simulink model "Controls"  (R2024b)
settings: Solver=VariableStepAuto  StartTime=0.0  StopTime=10.0  RelTol=1e-3
settings Model: Creator=Rayhaan T  LastModifiedBy=Rayhaan T

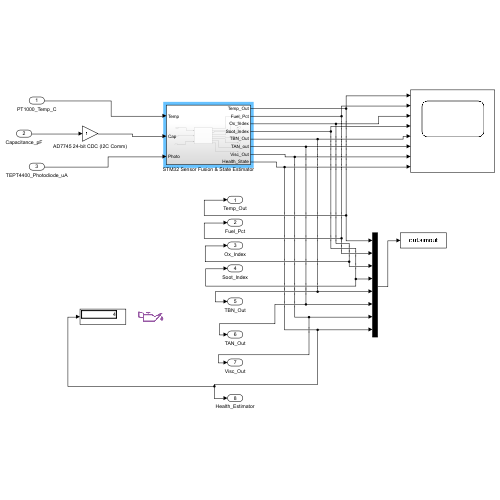
[thumbnail: Simulink's stored preview of the top-level diagram]
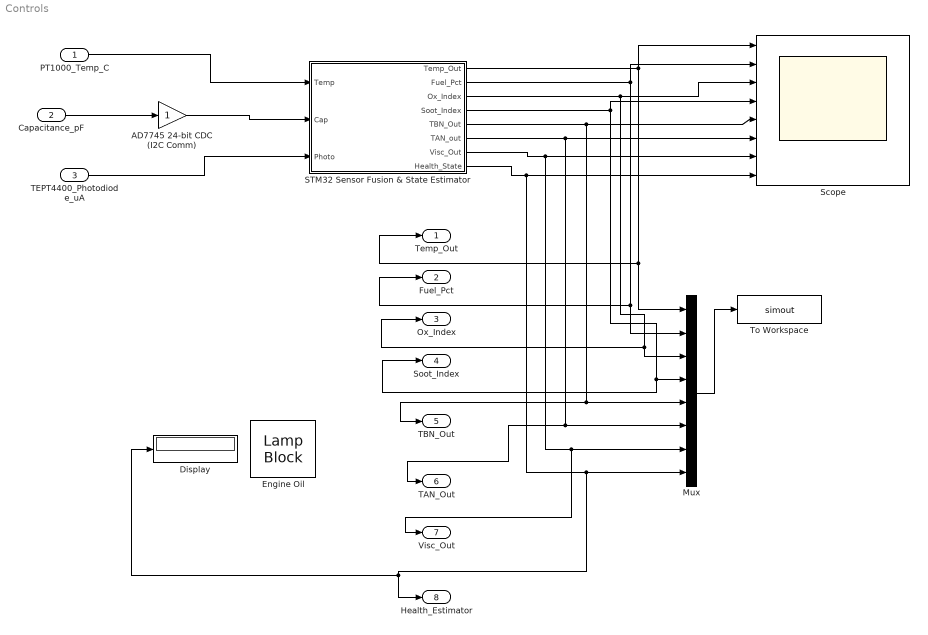
== system Controls ==
  PT1000_Temp_C : Inport
  Capacitance_pF : Inport  Port=2
  TEPT4400_Photodiode_uA : Inport  Port=3
  AD7745 24-bit CDC (I2C Comm) : Gain
  Display : Display
  Engine Oil : LampBlock  LabelPosition=Hide  Icon=EngineOil
  Mux : Mux  Inputs=8
  STM32 Sensor Fusion & State Estimator : Subsystem
  Scope : Scope  NumInputPorts=8
  To Workspace : ToWorkspace  VariableName=simout  SaveFormat=Timeseries  SampleTime=-1
  Temp_Out : Outport
  Fuel_Pct : Outport  Port=2
  Ox_Index : Outport  Port=3
  Soot_Index : Outport  Port=4
  TBN_Out : Outport  Port=5
  TAN_Out : Outport  Port=6
  Visc_Out : Outport  Port=7
  Health_Estimator : Outport  Port=8
  wires:
  Capacitance_pF/1 -> AD7745 24-bit CDC (I2C Comm)/1
  PT1000_Temp_C/1 -> STM32 Sensor Fusion & State Estimator/1(Temp)
  TEPT4400_Photodiode_uA/1 -> STM32 Sensor Fusion & State Estimator/3(Photo)
  STM32 Sensor Fusion & State Estimator/1(Temp_Out) -> Temp_Out/1, Mux/1, Scope/1
  STM32 Sensor Fusion & State Estimator/2(Fuel_Pct) -> Fuel_Pct/1, Mux/2, Scope/2
  STM32 Sensor Fusion & State Estimator/4(Soot_Index) -> Soot_Index/1, Mux/4, Scope/4
  STM32 Sensor Fusion & State Estimator/3(Ox_Index) -> Ox_Index/1, Mux/3, Scope/3
  AD7745 24-bit CDC (I2C Comm)/1 -> STM32 Sensor Fusion & State Estimator/2(Cap)
  Mux/1 -> To Workspace/1
  STM32 Sensor Fusion & State Estimator/5(TBN_Out) -> Mux/5, TBN_Out/1, Scope/5
  STM32 Sensor Fusion & State Estimator/6(TAN_out) -> Mux/6, TAN_Out/1, Scope/6
  STM32 Sensor Fusion & State Estimator/7(Visc_Out) -> Visc_Out/1, Mux/7, Scope/7
  STM32 Sensor Fusion & State Estimator/8(Health_State) -> Display/1, Health_Estimator/1, Mux/8, Scope/8

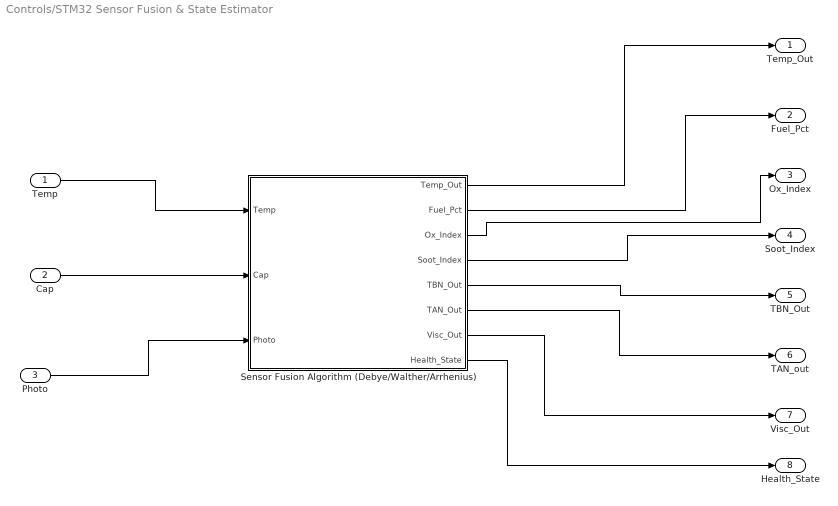
== system Controls/STM32 Sensor Fusion & State Estimator ==
  Temp : Inport
  Cap : Inport  Port=2
  Photo : Inport  Port=3
  Sensor Fusion Algorithm (Debye/Walther/Arrhenius) : MATLAB Function  TreatAsAtomicUnit=on
  Temp_Out : Outport
  Fuel_Pct : Outport  Port=2
  Ox_Index : Outport  Port=3
  Soot_Index : Outport  Port=4
  TBN_Out : Outport  Port=5
  TAN_out : Outport  Port=6
  Visc_Out : Outport  Port=7
  Health_State : Outport  Port=8
  wires:
  Temp/1 -> Sensor Fusion Algorithm (Debye/Walther/Arrhenius)/1(Temp)
  Cap/1 -> Sensor Fusion Algorithm (Debye/Walther/Arrhenius)/2(Cap)
  Photo/1 -> Sensor Fusion Algorithm (Debye/Walther/Arrhenius)/3(Photo)
  Sensor Fusion Algorithm (Debye/Walther/Arrhenius)/1(Temp_Out) -> Temp_Out/1
  Sensor Fusion Algorithm (Debye/Walther/Arrhenius)/2(Fuel_Pct) -> Fuel_Pct/1
  Sensor Fusion Algorithm (Debye/Walther/Arrhenius)/3(Ox_Index) -> Ox_Index/1
  Sensor Fusion Algorithm (Debye/Walther/Arrhenius)/4(Soot_Index) -> Soot_Index/1
  Sensor Fusion Algorithm (Debye/Walther/Arrhenius)/5(TBN_Out) -> TBN_Out/1
  Sensor Fusion Algorithm (Debye/Walther/Arrhenius)/6(TAN_Out) -> TAN_out/1
  Sensor Fusion Algorithm (Debye/Walther/Arrhenius)/7(Visc_Out) -> Visc_Out/1
  Sensor Fusion Algorithm (Debye/Walther/Arrhenius)/8(Health_State) -> Health_State/1

== matlab function Controls/STM32 Sensor Fusion & State Estimator/Sensor Fusion Algorithm (Debye//Walther//Arrhenius) ==
  data: Temp input; Temp_Out output; Fuel_Pct output; Ox_Index output; Soot_Index output; Cap input; Photo input; TBN_Out output; TAN_Out output; Visc_Out output; Health_State output
function [Temp_Out, Fuel_Pct, Ox_Index, Soot_Index, TBN_Out, TAN_Out, Visc_Out, Health_State] = fcn(Temp, Cap, Photo)
    % --- HARDCODED BASELINES FOR SAE 15W-40 ---
    Base_Cap = 15.0;     % Nominal fresh oil capacitance (pF)
    Base_Visc = 105.0;   % Kinematic Viscosity at 40C (cSt)
    TAN_Init = 2.0;      % Fresh oil Total Acid Number (mg KOH/g)
    TBN_Init = 12.0;     % Fresh oil Total Base Number (mg KOH/g)
    
    % --- 1. TEMPERATURE COMPENSATION & ARRHENIUS RATE ---
    % Expected capacitance drops slightly as temp increases (density thins)
    Expected_Cap = Base_Cap - (0.01 * (Temp - 40)); 
    
    % Oxidation rate doubles every 10 degrees over 80C
    Ox_Rate = 1.0; 
    if Temp > 80
        Ox_Rate = 2 ^ ((Temp - 80) / 10.0);
    end
    
    % --- 2. POLARITY INDEX (CAPACITANCE DELTA) ---
    Delta_C = Cap - Expected_Cap;
    
    % --- 3. OPTICAL DENSITY (SOOT / SLUDGE) ---
    % Prevent log of zero or negative numbers
    if Photo < 1.0
        Photo = 1.0; 
    end
    Optical_Density = log10(300.0 / Photo);
    
    % --- 4. SENSOR FUSION ENGINE (Solving for unmeasured variables) ---
    Fuel_Fraction = 0.0;
    Oxidation_Factor = 0.0;
    
    if Delta_C < -0.5 
        % Capacitance dropped: Non-polar fuel dilution is dominating
        Fuel_Fraction = abs(Delta_C) * 0.05; 
    elseif Delta_C > 0.5
        % Capacitance increased: Polar oxidation products are building up
        Oxidation_Factor = Delta_C * 0.1 * Ox_Rate;
    end
    
    % THE V-CURVE TIE-BREAKER (If Cap seems 'normal' but oil is pitch black)
    if (abs(Delta_C) <= 0.5) && (Optical_Density > 0.6)
        Fuel_Fraction = 0.10;   % Hidden heavy fuel dilution
        Oxidation_Factor = 2.0; % Hidden heavy oxidation sludge
    end
    
    % --- 5. FORMAT OUTPUTS FOR THE 8-CHANNEL DAQ ---
    Temp_Out = Temp;                        % Parameter 1: Temperature (C)
    Fuel_Pct = Fuel_Fraction * 100.0;       % Parameter 2: Fuel Dilution (%)
    Ox_Index = Oxidation_Factor * 100.0;    % Parameter 3: Oxidation Index (0-100)
    Soot_Index = Optical_Density * 100.0;   % Parameter 4: Soot/Sludge Index (0-100)
    
    % Acid / Base Math
    TAN_Out = TAN_Init + (Oxidation_Factor * 1.5); % Advanced Metric 1: TAN
    TBN_Out = TBN_Init - 1.2 * (TAN_Out - TAN_Init); % Parameter 5: TBN
    if TBN_Out < 2.0
        TBN_Out = 2.0; % Failsafe floor
    end
    
    % Viscosity V-Curve Math
    Visc_Drop = Fuel_Fraction * 40.0; 
    Visc_Spike = Oxidation_Factor * 25.0;
    Visc_Out = Base_Visc - Visc_Drop + Visc_Spike; % Advanced Metric 2: Kinematic Viscosity
    
    % --- 6. HEALTH STATE DIAGNOSTICS MACHINE ---
    % 0 = Healthy, 1 = Fuel Warning, 2 = Heat/Ox Warning, 3 = Acid Critical, 4 = Sludge Critical
    Health_State = 0; % Default to Healthy
    
    if Fuel_Pct > 5.0 && Fuel_Pct <= 8.0
        Health_State = 1; % State 1: Fuel Leak creeping up
    elseif Ox_Index > 50.0 || Temp > 105.0
        Health_State = 2; % State 2: Running hot or heavy oxidation
    end
    
    % Critical Overrides (These trump the warnings)
    if TBN_Out < 5.0
        Health_State = 3; % State 3: TBN severely depleted. Corrosion imminent.
    elseif Soot_Index > 80.0 && Fuel_Pct > 8.0
        Health_State = 4; % State 4: The V-Curve Death Zone (Cancel-out effect)
    end
end
